simulink model "doc_lmseq"  (R2014a)
settings: Solver=ode45  StartTime=0.0  StopTime=inf  RelTol=1e-3
undefined symbols (not defined in the file or in its folder): commblksprivate, dfilt, Info, qammod
libraries: commchan3 x1, dsparch4 x1, commeq2 x1, commrandsrc2 x1, commdigbbndam3 x1, dspmtrx3 x1
settings Model: ExtModeAutoUpdateStatusClock=off  Creator=The MathWorks Inc.
settings DataIOCC: SignalLoggingSaveFormat=ModelDataLogs  SignalLoggingName=logsOut
settings OptimizationCC: ExpressionDepthLimit=2147483647  InitFltsAndDblsToZero=on
settings DebuggingCC: SaveWithParameterizedLinksMsg=none  UnderspecifiedInitializationDetection=Classic  CheckExecutionContextPreStartOutputMsg=on  CheckExecutionContextRuntimeOutputMsg=on  SignalResolutionControl=TryResolveAllWithWarning  SolverPrmCheckMsg=none  InheritedTsInSrcMsg=none  MultiTaskDSMMsg=warning  MultiTaskCondExecSysMsg=none  FcnCallInpInsideContextMsg=UseLocalSettings  StateNameClashWarn=warning  StrictBusMsg=None
settings HardwareCC: ProdHWDeviceType=Specified
settings ModelReferenceCC: UpdateModelReferenceTargets=IfOutOfDate
settings RTWCC: IncludeERTFirstTime=on
settings CodeAppCC: MangleLength=5
settings GRTTargetCC: TargetFcnLib=ansi_tfl_tmw.mat  CombineOutputUpdateFcns=off  GRTInterface=on

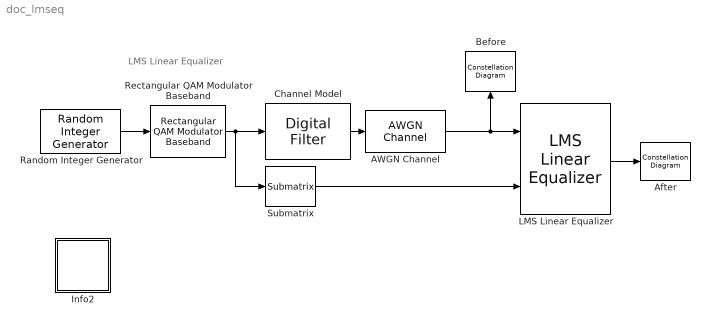
== system doc_lmseq ==
  note: LMS Linear Equalizer
  AWGN Channel : commchan3/AWGN Channel  InputProcessing=Columns as channels (frame based)  seed=67  noiseMode="Signal to noise ratio  (SNR)"  EbNodB=10  EsNodB=10  SNRdB=40  bitsPerSym=1  Ps=1  Tsym=1  variance=1
  After : ConstellationDiagram  Tag=ScatterPlot
  Before : ConstellationDiagram  Tag=ScatterPlot
  Channel Model : dsparch4/Digital Filter  TypePopup=FIR (all zeros)  IIRFiltStruct=Direct form I transposed  AllPoleFiltStruct=Direct form transposed  FIRFiltStruct=Direct form transposed  CoeffSource=Specify via dialog  NumCoeffs=[1 -.3 .1 .2j]  DenCoeffs=[1 0.1]  BiQuadCoeffs=[1 0.3 0.4 1 0.1 0.2]  LatticeCoeffs=[0.2 0.4]  denIgnore=on  FiltPerSampPopup=One filter per frame  IC=0  ICnum=0  ICden=0  roundingMode=Floor  overflowMode=off  ScaleValues=1  scaleValueFracLength=14  stageInFracLength=15  stageOutFracLength=15  FilterSource=Specify via dialog  dfiltObjectName=dfilt.dffir([1 2 1])  InputProcessing=Columns as channels (frame based)
  Info2 : Subsystem  AncestorBlock=commblksprivate/Info  mask(Info){}
      settings: OpenFcn=helpview([docroot '/toolbox/comm/comm.map'], 'doc_lmseq')
      mask Display: disp('Info')
  LMS Linear Equalizer : commeq2/LMS Linear  Equalizer  nTaps=6  nSamp=1  sigConst=qammod([0:15],16)  delay=2  stepSize=0.01  leakage=1  initWeights=0  mode=off  outErr=off  outWeights=off
  Random Integer Generator : commrandsrc2/Random Integer Generator  mul=16  seed=12345  Ts=1/1000  frameBased=on  sampPerFrame=1000  orient=off  outDataType=double
  Rectangular QAM Modulator Baseband : commdigbbndam3/Rectangular QAM Modulator Baseband  M=16  InType=Integer  Enc=Binary  Mapping=[0:15]  PowType=Average Power  MinDist=2  AvgPow=1  PeakPow=1  Ph=0  outDtype=double  outWordLen=16  outUDDataType=sfix(16)  outFracLenMode=Best precision  outFracLen=15
  Submatrix : dspmtrx3/Submatrix  RowSpan=Range of rows  RowStartMode=First  RowStartIndex=1  RowEndMode=Index  RowEndIndex=100  ColSpan=Range of columns  ColStartMode=First  ColStartIndex=1  ColEndMode=Last  ColEndIndex=1
  wires:
  Rectangular QAM Modulator Baseband/1 -> Submatrix/1, Channel Model/1
  Random Integer Generator/1 -> Rectangular QAM Modulator Baseband/1
  Channel Model/1 -> AWGN Channel/1
  LMS Linear Equalizer/1 -> After/1
  Submatrix/1 -> LMS Linear Equalizer/2
  AWGN Channel/1 -> LMS Linear Equalizer/1, Before/1

== system doc_lmseq/Info2 ==
